simulink model "gm_FP_sub"  (R2023a)
settings: Solver=FixedStepAuto  StartTime=0.0  StopTime=T  RelTol=1e-3  EnableMultiTasking=on
undefined symbols (not defined in the file or in its folder): Ts
libraries: My_FI_Operations x114, simulink x1
(part 1 of 2)
settings Model: Creator=kavru  LastModifiedBy=kolbe
settings OptimizationCC: BlockReduction=off  ConditionallyExecuteInputs=off
settings DebuggingCC: SignalRangeChecking=warning  InheritedTsInSrcMsg=none  SingleTaskRateTransMsg=error  UnconnectedInputMsg=warning  UnconnectedOutputMsg=warning  UnconnectedLineMsg=warning
settings ModelReferenceCC: EnableRefExpFcnMdlSchedulingChecks=on
settings RTWCC: DLArmComputeVersion=19.05

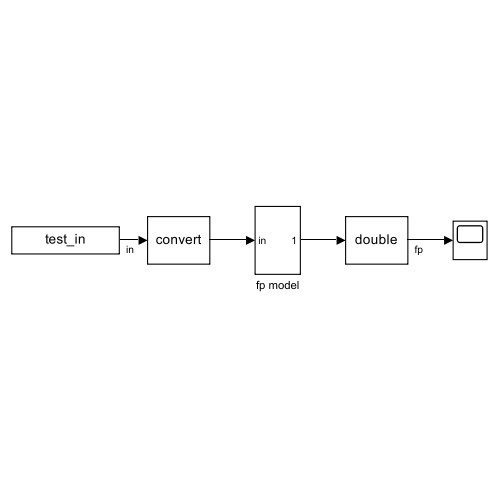
[thumbnail: Simulink's stored preview of the top-level diagram]
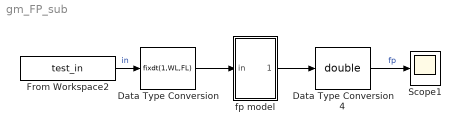
== system gm_FP_sub ==
  Data Type Conversion : DataTypeConversion  OutDataTypeStr=fixdt(1,WL,FL)  RndMeth=Nearest
  Data Type Conversion4 : DataTypeConversion  OutDataTypeStr=double  RndMeth=Nearest  SaturateOnIntegerOverflow=off
  From Workspace2 : FromWorkspace  VariableName=test_in  OutDataTypeStr=double  SampleTime=Ts
  Scope1 : Scope
  fp model : Subsystem
  wires:
  Data Type Conversion4/1 -> Scope1/1  "fp"
  Data Type Conversion/1 -> fp model/1(in)
  fp model/1(Out1) -> Data Type Conversion4/1
  From Workspace2/1 -> Data Type Conversion/1  "in"

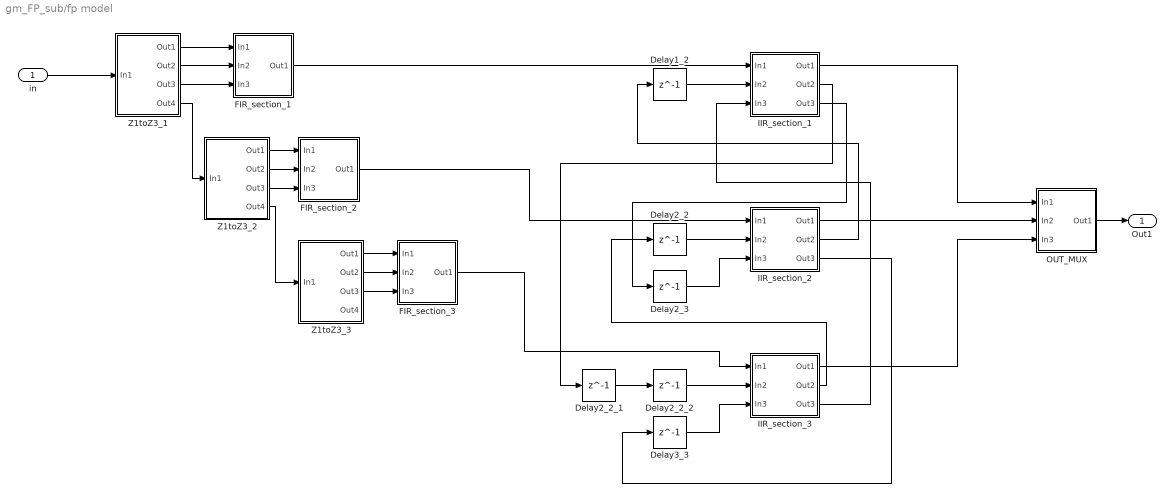
== system gm_FP_sub/fp model ==
  in : Inport
  Delay1_2 : Delay  DelayLength=1  SampleTime=3*Ts
  Delay2_2 : Delay  DelayLength=1  SampleTime=3*Ts
  Delay2_2_1 : Delay  DelayLength=1  SampleTime=3*Ts
  Delay2_2_2 : Delay  DelayLength=1  SampleTime=3*Ts
  Delay2_3 : Delay  DelayLength=1  SampleTime=3*Ts
  Delay3_3 : Delay  DelayLength=1  SampleTime=3*Ts
  FIR_section_1 : Subsystem
  FIR_section_2 : Subsystem
  FIR_section_3 : Subsystem
  IIR_section_1 : Subsystem
  IIR_section_2 : Subsystem
  IIR_section_3 : Subsystem
  OUT_MUX : Subsystem
  Z1toZ3_1 : Subsystem
  Z1toZ3_2 : Subsystem
  Z1toZ3_3 : Subsystem
  Out1 : Outport
  wires:
  IIR_section_1/2(Out2) -> Delay2_2_1/1
  Delay2_2_1/1 -> Delay2_2_2/1
  IIR_section_3/2(Out2) -> Delay2_2/1
  IIR_section_3/1(Out1) -> OUT_MUX/3(In3)
  IIR_section_3/3(Out3) -> IIR_section_1/3(In3)
  FIR_section_3/1(Out1) -> IIR_section_3/1(In1)
  Delay3_3/1 -> IIR_section_3/3(In3)
  Delay2_2_2/1 -> IIR_section_3/2(In2)
  IIR_section_2/3(Out3) -> Delay3_3/1
  IIR_section_2/2(Out2) -> Delay1_2/1
  IIR_section_2/1(Out1) -> OUT_MUX/2(In2)
  Delay2_2/1 -> IIR_section_2/2(In2)
  Delay2_3/1 -> IIR_section_2/3(In3)
  FIR_section_2/1(Out1) -> IIR_section_2/1(In1)
  IIR_section_1/3(Out3) -> Delay2_3/1
  IIR_section_1/1(Out1) -> OUT_MUX/1(In1)
  Delay1_2/1 -> IIR_section_1/2(In2)
  FIR_section_1/1(Out1) -> IIR_section_1/1(In1)
  OUT_MUX/1(Out1) -> Out1/1
  Z1toZ3_3/3(Out3) -> FIR_section_3/3(In3)
  Z1toZ3_3/2(Out2) -> FIR_section_3/2(In2)
  Z1toZ3_3/1(Out1) -> FIR_section_3/1(In1)
  Z1toZ3_2/3(Out3) -> FIR_section_2/3(In3)
  Z1toZ3_2/2(Out2) -> FIR_section_2/2(In2)
  Z1toZ3_2/1(Out1) -> FIR_section_2/1(In1)
  Z1toZ3_1/3(Out3) -> FIR_section_1/3(In3)
  Z1toZ3_1/2(Out2) -> FIR_section_1/2(In2)
  Z1toZ3_1/1(Out1) -> FIR_section_1/1(In1)
  Z1toZ3_2/4(Out4) -> Z1toZ3_3/1(In1)
  Z1toZ3_1/4(Out4) -> Z1toZ3_2/1(In1)
  in/1 -> Z1toZ3_1/1(In1)

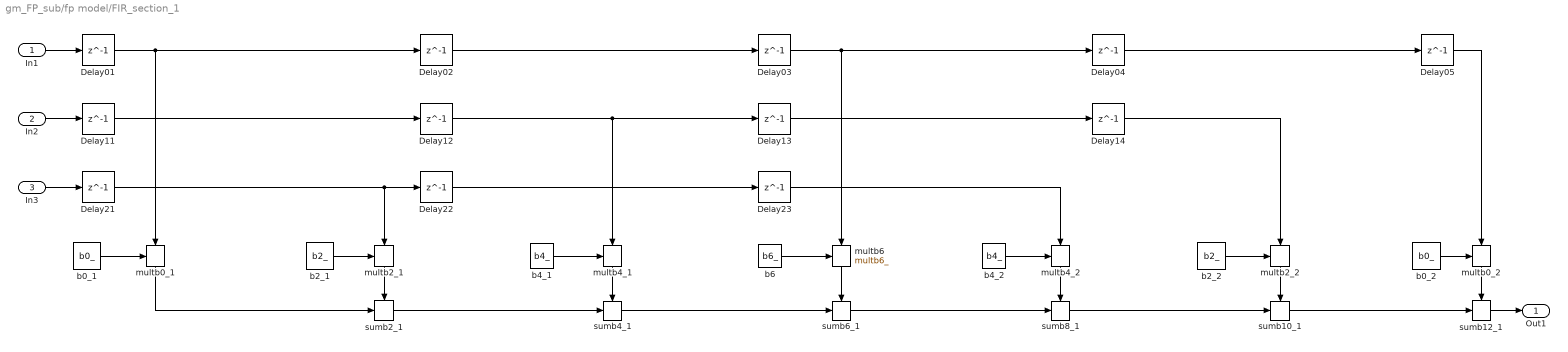
== system gm_FP_sub/fp model/FIR_section_1 ==
  In1 : Inport
  In2 : Inport  Port=2
  In3 : Inport  Port=3
  Delay01 : Delay  DelayLength=1  SampleTime=3*Ts
  Delay02 : Delay  DelayLength=1  SampleTime=3*Ts
  Delay03 : Delay  DelayLength=1  SampleTime=3*Ts
  Delay04 : Delay  DelayLength=1  SampleTime=3*Ts
  Delay05 : Delay  DelayLength=1  SampleTime=3*Ts
  Delay{11..14,21..23} (7 alike) : Delay  DelayLength=1  SampleTime=3*Ts
  b0_1 : My_FI_Operations/b0_  SystemSampleTime=-1  VariantActivationTime=update diagram  Latency=0  AutoFrameSizeCalculation=off
  b0_2 : My_FI_Operations/b0_  SystemSampleTime=-1  VariantActivationTime=update diagram  Latency=0  AutoFrameSizeCalculation=off
  b2_1 : My_FI_Operations/b2_  SystemSampleTime=-1  VariantActivationTime=update diagram  Latency=0  AutoFrameSizeCalculation=off
  b2_2 : My_FI_Operations/b2_  SystemSampleTime=-1  VariantActivationTime=update diagram  Latency=0  AutoFrameSizeCalculation=off
  b4_1 : My_FI_Operations/b4_  SystemSampleTime=-1  VariantActivationTime=update diagram  Latency=0  AutoFrameSizeCalculation=off
  b4_2 : My_FI_Operations/b4_  SystemSampleTime=-1  VariantActivationTime=update diagram  Latency=0  AutoFrameSizeCalculation=off
  b6 : My_FI_Operations/b6_  SystemSampleTime=-1  VariantActivationTime=update diagram  Latency=0  AutoFrameSizeCalculation=off
  multb0_1 : My_FI_Operations/multb0_  SystemSampleTime=-1  VariantActivationTime=update diagram  Latency=0  AutoFrameSizeCalculation=off
      settings: PortSchema="{\"entries\":[{\"content\":{\"sides\":[{\"content\":{\"connectorIds\":[\"In1\"]},\"type\":\"ConnectorPlacement.EquallySpacedRectSide\",\"uuid\":\"20461ecc-945a-453b-bec8-f18bcbd4d7ca\"},{\"content\":{\"connectorIds\":[],\"side\":\"RIGHT\"},\"type\":\"ConnectorPlacement.EquallySpacedRectSide\",\"uuid\":\"a806ae65-26a1-4387-823f-a90265b6c751\"},{\"content\":{\"connectorIds\":[\"In2\"],\"side\":\"TOP\"},\"type\":\"ConnectorPlacement.EquallySpacedRectSide\",\"uuid\":\"faa34e1a-fdc6-4b39-b604-acf00955d353\"},{\"content\":{\"connectorIds\":[\"Out1\"],\"side\":\"BOTTOM\"},\"type\":\"ConnectorPlacement.EquallySpacedRectSide\",\"uuid\":\"6d48c7d1-ec45-4610-bf5d-3af7cf103011\"}]},\"type\":\"ConnectorPlacement.EquallySpacedConnector\",\"uuid\":\"f3c21808-e34e-4785-8275-0070ba5b450f\"}],\"packageUris\":[\"http://schema.mathworks.com/mf0/Connector/R2020b\"],\"version\":\"1.0\"}"
  multb0_2 : My_FI_Operations/multb0_  SystemSampleTime=-1  VariantActivationTime=update diagram  Latency=0  AutoFrameSizeCalculation=off
      settings: PortSchema="{\"entries\":[{\"content\":{\"sides\":[{\"content\":{\"connectorIds\":[\"In1\"]},\"type\":\"ConnectorPlacement.EquallySpacedRectSide\",\"uuid\":\"20461ecc-945a-453b-bec8-f18bcbd4d7ca\"},{\"content\":{\"connectorIds\":[],\"side\":\"RIGHT\"},\"type\":\"ConnectorPlacement.EquallySpacedRectSide\",\"uuid\":\"a806ae65-26a1-4387-823f-a90265b6c751\"},{\"content\":{\"connectorIds\":[\"In2\"],\"side\":\"TOP\"},\"type\":\"ConnectorPlacement.EquallySpacedRectSide\",\"uuid\":\"faa34e1a-fdc6-4b39-b604-acf00955d353\"},{\"content\":{\"connectorIds\":[\"Out1\"],\"side\":\"BOTTOM\"},\"type\":\"ConnectorPlacement.EquallySpacedRectSide\",\"uuid\":\"6d48c7d1-ec45-4610-bf5d-3af7cf103011\"}]},\"type\":\"ConnectorPlacement.EquallySpacedConnector\",\"uuid\":\"f3c21808-e34e-4785-8275-0070ba5b450f\"}],\"packageUris\":[\"http://schema.mathworks.com/mf0/Connector/R2020b\"],\"version\":\"1.0\"}"
  multb2_1 : My_FI_Operations/multb2_  SystemSampleTime=-1  VariantActivationTime=update diagram  Latency=0  AutoFrameSizeCalculation=off
      settings: PortSchema="{\"entries\":[{\"content\":{\"sides\":[{\"content\":{\"connectorIds\":[\"In1\"]},\"type\":\"ConnectorPlacement.EquallySpacedRectSide\",\"uuid\":\"20461ecc-945a-453b-bec8-f18bcbd4d7ca\"},{\"content\":{\"connectorIds\":[],\"side\":\"RIGHT\"},\"type\":\"ConnectorPlacement.EquallySpacedRectSide\",\"uuid\":\"a806ae65-26a1-4387-823f-a90265b6c751\"},{\"content\":{\"connectorIds\":[\"In2\"],\"side\":\"TOP\"},\"type\":\"ConnectorPlacement.EquallySpacedRectSide\",\"uuid\":\"faa34e1a-fdc6-4b39-b604-acf00955d353\"},{\"content\":{\"connectorIds\":[\"Out1\"],\"side\":\"BOTTOM\"},\"type\":\"ConnectorPlacement.EquallySpacedRectSide\",\"uuid\":\"e1b0fef8-c153-494e-8ffe-3515e962a3c5\"}]},\"type\":\"ConnectorPlacement.EquallySpacedConnector\",\"uuid\":\"f3c21808-e34e-4785-8275-0070ba5b450f\"}],\"packageUris\":[\"http://schema.mathworks.com/mf0/Connector/R2020b\"],\"version\":\"1.0\"}"
  multb2_2 : My_FI_Operations/multb2_  SystemSampleTime=-1  VariantActivationTime=update diagram  Latency=0  AutoFrameSizeCalculation=off
      settings: PortSchema="{\"entries\":[{\"content\":{\"sides\":[{\"content\":{\"connectorIds\":[\"In1\"]},\"type\":\"ConnectorPlacement.EquallySpacedRectSide\",\"uuid\":\"20461ecc-945a-453b-bec8-f18bcbd4d7ca\"},{\"content\":{\"connectorIds\":[],\"side\":\"RIGHT\"},\"type\":\"ConnectorPlacement.EquallySpacedRectSide\",\"uuid\":\"a806ae65-26a1-4387-823f-a90265b6c751\"},{\"content\":{\"connectorIds\":[\"In2\"],\"side\":\"TOP\"},\"type\":\"ConnectorPlacement.EquallySpacedRectSide\",\"uuid\":\"faa34e1a-fdc6-4b39-b604-acf00955d353\"},{\"content\":{\"connectorIds\":[\"Out1\"],\"side\":\"BOTTOM\"},\"type\":\"ConnectorPlacement.EquallySpacedRectSide\",\"uuid\":\"e1b0fef8-c153-494e-8ffe-3515e962a3c5\"}]},\"type\":\"ConnectorPlacement.EquallySpacedConnector\",\"uuid\":\"f3c21808-e34e-4785-8275-0070ba5b450f\"}],\"packageUris\":[\"http://schema.mathworks.com/mf0/Connector/R2020b\"],\"version\":\"1.0\"}"
  multb4_1 : My_FI_Operations/multb4_  SystemSampleTime=-1  VariantActivationTime=update diagram  Latency=0  AutoFrameSizeCalculation=off
      settings: PortSchema="{\"entries\":[{\"content\":{\"sides\":[{\"content\":{\"connectorIds\":[\"In1\"]},\"type\":\"ConnectorPlacement.EquallySpacedRectSide\",\"uuid\":\"20461ecc-945a-453b-bec8-f18bcbd4d7ca\"},{\"content\":{\"connectorIds\":[],\"side\":\"RIGHT\"},\"type\":\"ConnectorPlacement.EquallySpacedRectSide\",\"uuid\":\"a806ae65-26a1-4387-823f-a90265b6c751\"},{\"content\":{\"connectorIds\":[\"In2\"],\"side\":\"TOP\"},\"type\":\"ConnectorPlacement.EquallySpacedRectSide\",\"uuid\":\"faa34e1a-fdc6-4b39-b604-acf00955d353\"},{\"content\":{\"connectorIds\":[\"Out1\"],\"side\":\"BOTTOM\"},\"type\":\"ConnectorPlacement.EquallySpacedRectSide\",\"uuid\":\"234e609c-6b95-41af-91dd-8a06091f2e10\"}]},\"type\":\"ConnectorPlacement.EquallySpacedConnector\",\"uuid\":\"f3c21808-e34e-4785-8275-0070ba5b450f\"}],\"packageUris\":[\"http://schema.mathworks.com/mf0/Connector/R2020b\"],\"version\":\"1.0\"}"
  multb4_2 : My_FI_Operations/multb4_  SystemSampleTime=-1  VariantActivationTime=update diagram  Latency=0  AutoFrameSizeCalculation=off
      settings: PortSchema="{\"entries\":[{\"content\":{\"sides\":[{\"content\":{\"connectorIds\":[\"In1\"]},\"type\":\"ConnectorPlacement.EquallySpacedRectSide\",\"uuid\":\"20461ecc-945a-453b-bec8-f18bcbd4d7ca\"},{\"content\":{\"connectorIds\":[],\"side\":\"RIGHT\"},\"type\":\"ConnectorPlacement.EquallySpacedRectSide\",\"uuid\":\"a806ae65-26a1-4387-823f-a90265b6c751\"},{\"content\":{\"connectorIds\":[\"In2\"],\"side\":\"TOP\"},\"type\":\"ConnectorPlacement.EquallySpacedRectSide\",\"uuid\":\"faa34e1a-fdc6-4b39-b604-acf00955d353\"},{\"content\":{\"connectorIds\":[\"Out1\"],\"side\":\"BOTTOM\"},\"type\":\"ConnectorPlacement.EquallySpacedRectSide\",\"uuid\":\"234e609c-6b95-41af-91dd-8a06091f2e10\"}]},\"type\":\"ConnectorPlacement.EquallySpacedConnector\",\"uuid\":\"f3c21808-e34e-4785-8275-0070ba5b450f\"}],\"packageUris\":[\"http://schema.mathworks.com/mf0/Connector/R2020b\"],\"version\":\"1.0\"}"
  multb6 : My_FI_Operations/multb6_  SystemSampleTime=-1  VariantActivationTime=update diagram  Latency=0  AutoFrameSizeCalculation=off
      settings: PortSchema="{\"entries\":[{\"content\":{\"sides\":[{\"content\":{\"connectorIds\":[\"In1\"]},\"type\":\"ConnectorPlacement.EquallySpacedRectSide\",\"uuid\":\"20461ecc-945a-453b-bec8-f18bcbd4d7ca\"},{\"content\":{\"connectorIds\":[],\"side\":\"RIGHT\"},\"type\":\"ConnectorPlacement.EquallySpacedRectSide\",\"uuid\":\"a806ae65-26a1-4387-823f-a90265b6c751\"},{\"content\":{\"connectorIds\":[\"In2\"],\"side\":\"TOP\"},\"type\":\"ConnectorPlacement.EquallySpacedRectSide\",\"uuid\":\"faa34e1a-fdc6-4b39-b604-acf00955d353\"},{\"content\":{\"connectorIds\":[\"Out1\"],\"side\":\"BOTTOM\"},\"type\":\"ConnectorPlacement.EquallySpacedRectSide\",\"uuid\":\"31f2fa17-ae8c-4166-97ac-b63529612348\"}]},\"type\":\"ConnectorPlacement.EquallySpacedConnector\",\"uuid\":\"f3c21808-e34e-4785-8275-0070ba5b450f\"}],\"packageUris\":[\"http://schema.mathworks.com/mf0/Connector/R2020b\"],\"version\":\"1.0\"}"
  sumb10_1 : My_FI_Operations/sumb10_  SystemSampleTime=-1  VariantActivationTime=update diagram  Latency=0  AutoFrameSizeCalculation=off
      settings: PortSchema="{\"entries\":[{\"content\":{\"sides\":[{\"content\":{\"connectorIds\":[\"In1\"]},\"type\":\"ConnectorPlacement.EquallySpacedRectSide\",\"uuid\":\"20461ecc-945a-453b-bec8-f18bcbd4d7ca\"},{\"content\":{\"connectorIds\":[\"Out1\"],\"side\":\"RIGHT\"},\"type\":\"ConnectorPlacement.EquallySpacedRectSide\",\"uuid\":\"a806ae65-26a1-4387-823f-a90265b6c751\"},{\"content\":{\"connectorIds\":[\"In2\"],\"side\":\"TOP\"},\"type\":\"ConnectorPlacement.EquallySpacedRectSide\",\"uuid\":\"faa34e1a-fdc6-4b39-b604-acf00955d353\"}]},\"type\":\"ConnectorPlacement.EquallySpacedConnector\",\"uuid\":\"f3c21808-e34e-4785-8275-0070ba5b450f\"}],\"packageUris\":[\"http://schema.mathworks.com/mf0/Connector/R2020b\"],\"version\":\"1.0\"}"
  sumb12_1 : My_FI_Operations/sumb12_  SystemSampleTime=-1  VariantActivationTime=update diagram  Latency=0  AutoFrameSizeCalculation=off
      settings: PortSchema="{\"entries\":[{\"content\":{\"sides\":[{\"content\":{\"connectorIds\":[\"In1\"]},\"type\":\"ConnectorPlacement.EquallySpacedRectSide\",\"uuid\":\"20461ecc-945a-453b-bec8-f18bcbd4d7ca\"},{\"content\":{\"connectorIds\":[\"Out1\"],\"side\":\"RIGHT\"},\"type\":\"ConnectorPlacement.EquallySpacedRectSide\",\"uuid\":\"a806ae65-26a1-4387-823f-a90265b6c751\"},{\"content\":{\"connectorIds\":[\"In2\"],\"side\":\"TOP\"},\"type\":\"ConnectorPlacement.EquallySpacedRectSide\",\"uuid\":\"faa34e1a-fdc6-4b39-b604-acf00955d353\"}]},\"type\":\"ConnectorPlacement.EquallySpacedConnector\",\"uuid\":\"f3c21808-e34e-4785-8275-0070ba5b450f\"}],\"packageUris\":[\"http://schema.mathworks.com/mf0/Connector/R2020b\"],\"version\":\"1.0\"}"
  sumb2_1 : My_FI_Operations/sumb2_  SystemSampleTime=-1  VariantActivationTime=update diagram  Latency=0  AutoFrameSizeCalculation=off
      settings: PortSchema="{\"entries\":[{\"content\":{\"sides\":[{\"content\":{\"connectorIds\":[\"In1\"]},\"type\":\"ConnectorPlacement.EquallySpacedRectSide\",\"uuid\":\"20461ecc-945a-453b-bec8-f18bcbd4d7ca\"},{\"content\":{\"connectorIds\":[\"Out1\"],\"side\":\"RIGHT\"},\"type\":\"ConnectorPlacement.EquallySpacedRectSide\",\"uuid\":\"a806ae65-26a1-4387-823f-a90265b6c751\"},{\"content\":{\"connectorIds\":[\"In2\"],\"side\":\"TOP\"},\"type\":\"ConnectorPlacement.EquallySpacedRectSide\",\"uuid\":\"faa34e1a-fdc6-4b39-b604-acf00955d353\"}]},\"type\":\"ConnectorPlacement.EquallySpacedConnector\",\"uuid\":\"f3c21808-e34e-4785-8275-0070ba5b450f\"}],\"packageUris\":[\"http://schema.mathworks.com/mf0/Connector/R2020b\"],\"version\":\"1.0\"}"
  sumb4_1 : My_FI_Operations/sumb4_  SystemSampleTime=-1  VariantActivationTime=update diagram  Latency=0  AutoFrameSizeCalculation=off
      settings: PortSchema="{\"entries\":[{\"content\":{\"sides\":[{\"content\":{\"connectorIds\":[\"In1\"]},\"type\":\"ConnectorPlacement.EquallySpacedRectSide\",\"uuid\":\"20461ecc-945a-453b-bec8-f18bcbd4d7ca\"},{\"content\":{\"connectorIds\":[\"Out1\"],\"side\":\"RIGHT\"},\"type\":\"ConnectorPlacement.EquallySpacedRectSide\",\"uuid\":\"a806ae65-26a1-4387-823f-a90265b6c751\"},{\"content\":{\"connectorIds\":[\"In2\"],\"side\":\"TOP\"},\"type\":\"ConnectorPlacement.EquallySpacedRectSide\",\"uuid\":\"faa34e1a-fdc6-4b39-b604-acf00955d353\"}]},\"type\":\"ConnectorPlacement.EquallySpacedConnector\",\"uuid\":\"f3c21808-e34e-4785-8275-0070ba5b450f\"}],\"packageUris\":[\"http://schema.mathworks.com/mf0/Connector/R2020b\"],\"version\":\"1.0\"}"
  sumb6_1 : My_FI_Operations/sumb6_  SystemSampleTime=-1  VariantActivationTime=update diagram  Latency=0  AutoFrameSizeCalculation=off
      settings: PortSchema="{\"entries\":[{\"content\":{\"sides\":[{\"content\":{\"connectorIds\":[\"In1\"]},\"type\":\"ConnectorPlacement.EquallySpacedRectSide\",\"uuid\":\"20461ecc-945a-453b-bec8-f18bcbd4d7ca\"},{\"content\":{\"connectorIds\":[\"Out1\"],\"side\":\"RIGHT\"},\"type\":\"ConnectorPlacement.EquallySpacedRectSide\",\"uuid\":\"a806ae65-26a1-4387-823f-a90265b6c751\"},{\"content\":{\"connectorIds\":[\"In2\"],\"side\":\"TOP\"},\"type\":\"ConnectorPlacement.EquallySpacedRectSide\",\"uuid\":\"faa34e1a-fdc6-4b39-b604-acf00955d353\"}]},\"type\":\"ConnectorPlacement.EquallySpacedConnector\",\"uuid\":\"f3c21808-e34e-4785-8275-0070ba5b450f\"}],\"packageUris\":[\"http://schema.mathworks.com/mf0/Connector/R2020b\"],\"version\":\"1.0\"}"
  sumb8_1 : My_FI_Operations/sumb8_  SystemSampleTime=-1  VariantActivationTime=update diagram  Latency=0  AutoFrameSizeCalculation=off
      settings: PortSchema="{\"entries\":[{\"content\":{\"sides\":[{\"content\":{\"connectorIds\":[\"In1\"]},\"type\":\"ConnectorPlacement.EquallySpacedRectSide\",\"uuid\":\"20461ecc-945a-453b-bec8-f18bcbd4d7ca\"},{\"content\":{\"connectorIds\":[\"Out1\"],\"side\":\"RIGHT\"},\"type\":\"ConnectorPlacement.EquallySpacedRectSide\",\"uuid\":\"a806ae65-26a1-4387-823f-a90265b6c751\"},{\"content\":{\"connectorIds\":[\"In2\"],\"side\":\"TOP\"},\"type\":\"ConnectorPlacement.EquallySpacedRectSide\",\"uuid\":\"faa34e1a-fdc6-4b39-b604-acf00955d353\"}]},\"type\":\"ConnectorPlacement.EquallySpacedConnector\",\"uuid\":\"f3c21808-e34e-4785-8275-0070ba5b450f\"}],\"packageUris\":[\"http://schema.mathworks.com/mf0/Connector/R2020b\"],\"version\":\"1.0\"}"
  Out1 : Outport
  wires:
  In1/1 -> Delay01/1
  sumb10_1/1 -> sumb12_1/1
  Delay04/1 -> Delay05/1
  multb2_2/1 -> sumb10_1/2
  In2/1 -> Delay11/1
  sumb2_1/1 -> sumb4_1/1
  Delay21/1 -> Delay22/1, multb2_1/2
  multb4_2/1 -> sumb8_1/2
  multb0_1/1 -> sumb2_1/1
  multb6/1 -> sumb6_1/2
  sumb12_1/1 -> Out1/1
  b4_1/1 -> multb4_1/1
  b2_1/1 -> multb2_1/1
  Delay05/1 -> multb0_2/2
  b6/1 -> multb6/1
  multb4_1/1 -> sumb4_1/2
  sumb4_1/1 -> sumb6_1/1
  Delay03/1 -> Delay04/1, multb6/2
  Delay02/1 -> Delay03/1
  Delay12/1 -> Delay13/1, multb4_1/2
  multb0_2/1 -> sumb12_1/2
  sumb8_1/1 -> sumb10_1/1
  b4_2/1 -> multb4_2/1
  b0_1/1 -> multb0_1/1
  b0_2/1 -> multb0_2/1
  Delay13/1 -> Delay14/1
  multb2_1/1 -> sumb2_1/2
  sumb6_1/1 -> sumb8_1/1
  Delay23/1 -> multb4_2/2
  b2_2/1 -> multb2_2/1
  Delay22/1 -> Delay23/1
  Delay14/1 -> multb2_2/2
  Delay01/1 -> Delay02/1, multb0_1/2
  Delay11/1 -> Delay12/1
  In3/1 -> Delay21/1

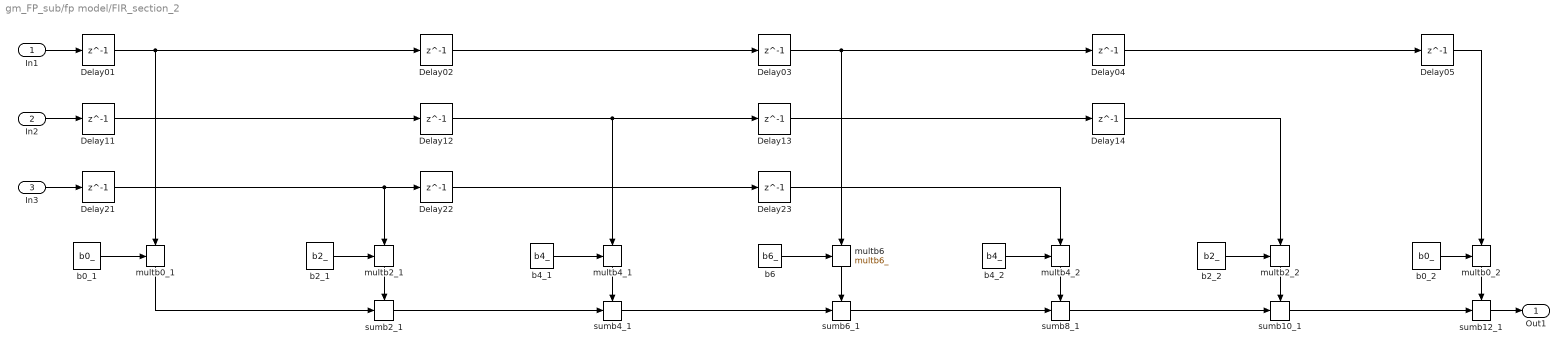
== system gm_FP_sub/fp model/FIR_section_2 ==
  In1 : Inport
  In2 : Inport  Port=2
  In3 : Inport  Port=3
  Delay01 : Delay  DelayLength=1  SampleTime=3*Ts
  Delay02 : Delay  DelayLength=1  SampleTime=3*Ts
  Delay03 : Delay  DelayLength=1  SampleTime=3*Ts
  Delay04 : Delay  DelayLength=1  SampleTime=3*Ts
  Delay05 : Delay  DelayLength=1  SampleTime=3*Ts
  Delay{11..14,21..23} (7 alike) : Delay  DelayLength=1  SampleTime=3*Ts
  b0_1 : My_FI_Operations/b0_  SystemSampleTime=-1  VariantActivationTime=update diagram  Latency=0  AutoFrameSizeCalculation=off
  b0_2 : My_FI_Operations/b0_  SystemSampleTime=-1  VariantActivationTime=update diagram  Latency=0  AutoFrameSizeCalculation=off
  b2_1 : My_FI_Operations/b2_  SystemSampleTime=-1  VariantActivationTime=update diagram  Latency=0  AutoFrameSizeCalculation=off
  b2_2 : My_FI_Operations/b2_  SystemSampleTime=-1  VariantActivationTime=update diagram  Latency=0  AutoFrameSizeCalculation=off
  b4_1 : My_FI_Operations/b4_  SystemSampleTime=-1  VariantActivationTime=update diagram  Latency=0  AutoFrameSizeCalculation=off
  b4_2 : My_FI_Operations/b4_  SystemSampleTime=-1  VariantActivationTime=update diagram  Latency=0  AutoFrameSizeCalculation=off
  b6 : My_FI_Operations/b6_  SystemSampleTime=-1  VariantActivationTime=update diagram  Latency=0  AutoFrameSizeCalculation=off
  multb0_1 : My_FI_Operations/multb0_  SystemSampleTime=-1  VariantActivationTime=update diagram  Latency=0  AutoFrameSizeCalculation=off
      settings: PortSchema="{\"entries\":[{\"content\":{\"sides\":[{\"content\":{\"connectorIds\":[\"In1\"]},\"type\":\"ConnectorPlacement.EquallySpacedRectSide\",\"uuid\":\"20461ecc-945a-453b-bec8-f18bcbd4d7ca\"},{\"content\":{\"connectorIds\":[],\"side\":\"RIGHT\"},\"type\":\"ConnectorPlacement.EquallySpacedRectSide\",\"uuid\":\"a806ae65-26a1-4387-823f-a90265b6c751\"},{\"content\":{\"connectorIds\":[\"In2\"],\"side\":\"TOP\"},\"type\":\"ConnectorPlacement.EquallySpacedRectSide\",\"uuid\":\"faa34e1a-fdc6-4b39-b604-acf00955d353\"},{\"content\":{\"connectorIds\":[\"Out1\"],\"side\":\"BOTTOM\"},\"type\":\"ConnectorPlacement.EquallySpacedRectSide\",\"uuid\":\"6d48c7d1-ec45-4610-bf5d-3af7cf103011\"}]},\"type\":\"ConnectorPlacement.EquallySpacedConnector\",\"uuid\":\"f3c21808-e34e-4785-8275-0070ba5b450f\"}],\"packageUris\":[\"http://schema.mathworks.com/mf0/Connector/R2020b\"],\"version\":\"1.0\"}"
  multb0_2 : My_FI_Operations/multb0_  SystemSampleTime=-1  VariantActivationTime=update diagram  Latency=0  AutoFrameSizeCalculation=off
      settings: PortSchema="{\"entries\":[{\"content\":{\"sides\":[{\"content\":{\"connectorIds\":[\"In1\"]},\"type\":\"ConnectorPlacement.EquallySpacedRectSide\",\"uuid\":\"20461ecc-945a-453b-bec8-f18bcbd4d7ca\"},{\"content\":{\"connectorIds\":[],\"side\":\"RIGHT\"},\"type\":\"ConnectorPlacement.EquallySpacedRectSide\",\"uuid\":\"a806ae65-26a1-4387-823f-a90265b6c751\"},{\"content\":{\"connectorIds\":[\"In2\"],\"side\":\"TOP\"},\"type\":\"ConnectorPlacement.EquallySpacedRectSide\",\"uuid\":\"faa34e1a-fdc6-4b39-b604-acf00955d353\"},{\"content\":{\"connectorIds\":[\"Out1\"],\"side\":\"BOTTOM\"},\"type\":\"ConnectorPlacement.EquallySpacedRectSide\",\"uuid\":\"6d48c7d1-ec45-4610-bf5d-3af7cf103011\"}]},\"type\":\"ConnectorPlacement.EquallySpacedConnector\",\"uuid\":\"f3c21808-e34e-4785-8275-0070ba5b450f\"}],\"packageUris\":[\"http://schema.mathworks.com/mf0/Connector/R2020b\"],\"version\":\"1.0\"}"
  multb2_1 : My_FI_Operations/multb2_  SystemSampleTime=-1  VariantActivationTime=update diagram  Latency=0  AutoFrameSizeCalculation=off
      settings: PortSchema="{\"entries\":[{\"content\":{\"sides\":[{\"content\":{\"connectorIds\":[\"In1\"]},\"type\":\"ConnectorPlacement.EquallySpacedRectSide\",\"uuid\":\"20461ecc-945a-453b-bec8-f18bcbd4d7ca\"},{\"content\":{\"connectorIds\":[],\"side\":\"RIGHT\"},\"type\":\"ConnectorPlacement.EquallySpacedRectSide\",\"uuid\":\"a806ae65-26a1-4387-823f-a90265b6c751\"},{\"content\":{\"connectorIds\":[\"In2\"],\"side\":\"TOP\"},\"type\":\"ConnectorPlacement.EquallySpacedRectSide\",\"uuid\":\"faa34e1a-fdc6-4b39-b604-acf00955d353\"},{\"content\":{\"connectorIds\":[\"Out1\"],\"side\":\"BOTTOM\"},\"type\":\"ConnectorPlacement.EquallySpacedRectSide\",\"uuid\":\"e1b0fef8-c153-494e-8ffe-3515e962a3c5\"}]},\"type\":\"ConnectorPlacement.EquallySpacedConnector\",\"uuid\":\"f3c21808-e34e-4785-8275-0070ba5b450f\"}],\"packageUris\":[\"http://schema.mathworks.com/mf0/Connector/R2020b\"],\"version\":\"1.0\"}"
  multb2_2 : My_FI_Operations/multb2_  SystemSampleTime=-1  VariantActivationTime=update diagram  Latency=0  AutoFrameSizeCalculation=off
      settings: PortSchema="{\"entries\":[{\"content\":{\"sides\":[{\"content\":{\"connectorIds\":[\"In1\"]},\"type\":\"ConnectorPlacement.EquallySpacedRectSide\",\"uuid\":\"20461ecc-945a-453b-bec8-f18bcbd4d7ca\"},{\"content\":{\"connectorIds\":[],\"side\":\"RIGHT\"},\"type\":\"ConnectorPlacement.EquallySpacedRectSide\",\"uuid\":\"a806ae65-26a1-4387-823f-a90265b6c751\"},{\"content\":{\"connectorIds\":[\"In2\"],\"side\":\"TOP\"},\"type\":\"ConnectorPlacement.EquallySpacedRectSide\",\"uuid\":\"faa34e1a-fdc6-4b39-b604-acf00955d353\"},{\"content\":{\"connectorIds\":[\"Out1\"],\"side\":\"BOTTOM\"},\"type\":\"ConnectorPlacement.EquallySpacedRectSide\",\"uuid\":\"e1b0fef8-c153-494e-8ffe-3515e962a3c5\"}]},\"type\":\"ConnectorPlacement.EquallySpacedConnector\",\"uuid\":\"f3c21808-e34e-4785-8275-0070ba5b450f\"}],\"packageUris\":[\"http://schema.mathworks.com/mf0/Connector/R2020b\"],\"version\":\"1.0\"}"
  multb4_1 : My_FI_Operations/multb4_  SystemSampleTime=-1  VariantActivationTime=update diagram  Latency=0  AutoFrameSizeCalculation=off
      settings: PortSchema="{\"entries\":[{\"content\":{\"sides\":[{\"content\":{\"connectorIds\":[\"In1\"]},\"type\":\"ConnectorPlacement.EquallySpacedRectSide\",\"uuid\":\"20461ecc-945a-453b-bec8-f18bcbd4d7ca\"},{\"content\":{\"connectorIds\":[],\"side\":\"RIGHT\"},\"type\":\"ConnectorPlacement.EquallySpacedRectSide\",\"uuid\":\"a806ae65-26a1-4387-823f-a90265b6c751\"},{\"content\":{\"connectorIds\":[\"In2\"],\"side\":\"TOP\"},\"type\":\"ConnectorPlacement.EquallySpacedRectSide\",\"uuid\":\"faa34e1a-fdc6-4b39-b604-acf00955d353\"},{\"content\":{\"connectorIds\":[\"Out1\"],\"side\":\"BOTTOM\"},\"type\":\"ConnectorPlacement.EquallySpacedRectSide\",\"uuid\":\"234e609c-6b95-41af-91dd-8a06091f2e10\"}]},\"type\":\"ConnectorPlacement.EquallySpacedConnector\",\"uuid\":\"f3c21808-e34e-4785-8275-0070ba5b450f\"}],\"packageUris\":[\"http://schema.mathworks.com/mf0/Connector/R2020b\"],\"version\":\"1.0\"}"
  multb4_2 : My_FI_Operations/multb4_  SystemSampleTime=-1  VariantActivationTime=update diagram  Latency=0  AutoFrameSizeCalculation=off
      settings: PortSchema="{\"entries\":[{\"content\":{\"sides\":[{\"content\":{\"connectorIds\":[\"In1\"]},\"type\":\"ConnectorPlacement.EquallySpacedRectSide\",\"uuid\":\"20461ecc-945a-453b-bec8-f18bcbd4d7ca\"},{\"content\":{\"connectorIds\":[],\"side\":\"RIGHT\"},\"type\":\"ConnectorPlacement.EquallySpacedRectSide\",\"uuid\":\"a806ae65-26a1-4387-823f-a90265b6c751\"},{\"content\":{\"connectorIds\":[\"In2\"],\"side\":\"TOP\"},\"type\":\"ConnectorPlacement.EquallySpacedRectSide\",\"uuid\":\"faa34e1a-fdc6-4b39-b604-acf00955d353\"},{\"content\":{\"connectorIds\":[\"Out1\"],\"side\":\"BOTTOM\"},\"type\":\"ConnectorPlacement.EquallySpacedRectSide\",\"uuid\":\"234e609c-6b95-41af-91dd-8a06091f2e10\"}]},\"type\":\"ConnectorPlacement.EquallySpacedConnector\",\"uuid\":\"f3c21808-e34e-4785-8275-0070ba5b450f\"}],\"packageUris\":[\"http://schema.mathworks.com/mf0/Connector/R2020b\"],\"version\":\"1.0\"}"
  multb6 : My_FI_Operations/multb6_  SystemSampleTime=-1  VariantActivationTime=update diagram  Latency=0  AutoFrameSizeCalculation=off
      settings: PortSchema="{\"entries\":[{\"content\":{\"sides\":[{\"content\":{\"connectorIds\":[\"In1\"]},\"type\":\"ConnectorPlacement.EquallySpacedRectSide\",\"uuid\":\"20461ecc-945a-453b-bec8-f18bcbd4d7ca\"},{\"content\":{\"connectorIds\":[],\"side\":\"RIGHT\"},\"type\":\"ConnectorPlacement.EquallySpacedRectSide\",\"uuid\":\"a806ae65-26a1-4387-823f-a90265b6c751\"},{\"content\":{\"connectorIds\":[\"In2\"],\"side\":\"TOP\"},\"type\":\"ConnectorPlacement.EquallySpacedRectSide\",\"uuid\":\"faa34e1a-fdc6-4b39-b604-acf00955d353\"},{\"content\":{\"connectorIds\":[\"Out1\"],\"side\":\"BOTTOM\"},\"type\":\"ConnectorPlacement.EquallySpacedRectSide\",\"uuid\":\"31f2fa17-ae8c-4166-97ac-b63529612348\"}]},\"type\":\"ConnectorPlacement.EquallySpacedConnector\",\"uuid\":\"f3c21808-e34e-4785-8275-0070ba5b450f\"}],\"packageUris\":[\"http://schema.mathworks.com/mf0/Connector/R2020b\"],\"version\":\"1.0\"}"
  sumb10_1 : My_FI_Operations/sumb10_  SystemSampleTime=-1  VariantActivationTime=update diagram  Latency=0  AutoFrameSizeCalculation=off
      settings: PortSchema="{\"entries\":[{\"content\":{\"sides\":[{\"content\":{\"connectorIds\":[\"In1\"]},\"type\":\"ConnectorPlacement.EquallySpacedRectSide\",\"uuid\":\"20461ecc-945a-453b-bec8-f18bcbd4d7ca\"},{\"content\":{\"connectorIds\":[\"Out1\"],\"side\":\"RIGHT\"},\"type\":\"ConnectorPlacement.EquallySpacedRectSide\",\"uuid\":\"a806ae65-26a1-4387-823f-a90265b6c751\"},{\"content\":{\"connectorIds\":[\"In2\"],\"side\":\"TOP\"},\"type\":\"ConnectorPlacement.EquallySpacedRectSide\",\"uuid\":\"faa34e1a-fdc6-4b39-b604-acf00955d353\"}]},\"type\":\"ConnectorPlacement.EquallySpacedConnector\",\"uuid\":\"f3c21808-e34e-4785-8275-0070ba5b450f\"}],\"packageUris\":[\"http://schema.mathworks.com/mf0/Connector/R2020b\"],\"version\":\"1.0\"}"
  sumb12_1 : My_FI_Operations/sumb12_  SystemSampleTime=-1  VariantActivationTime=update diagram  Latency=0  AutoFrameSizeCalculation=off
      settings: PortSchema="{\"entries\":[{\"content\":{\"sides\":[{\"content\":{\"connectorIds\":[\"In1\"]},\"type\":\"ConnectorPlacement.EquallySpacedRectSide\",\"uuid\":\"20461ecc-945a-453b-bec8-f18bcbd4d7ca\"},{\"content\":{\"connectorIds\":[\"Out1\"],\"side\":\"RIGHT\"},\"type\":\"ConnectorPlacement.EquallySpacedRectSide\",\"uuid\":\"a806ae65-26a1-4387-823f-a90265b6c751\"},{\"content\":{\"connectorIds\":[\"In2\"],\"side\":\"TOP\"},\"type\":\"ConnectorPlacement.EquallySpacedRectSide\",\"uuid\":\"faa34e1a-fdc6-4b39-b604-acf00955d353\"}]},\"type\":\"ConnectorPlacement.EquallySpacedConnector\",\"uuid\":\"f3c21808-e34e-4785-8275-0070ba5b450f\"}],\"packageUris\":[\"http://schema.mathworks.com/mf0/Connector/R2020b\"],\"version\":\"1.0\"}"
  sumb2_1 : My_FI_Operations/sumb2_  SystemSampleTime=-1  VariantActivationTime=update diagram  Latency=0  AutoFrameSizeCalculation=off
      settings: PortSchema="{\"entries\":[{\"content\":{\"sides\":[{\"content\":{\"connectorIds\":[\"In1\"]},\"type\":\"ConnectorPlacement.EquallySpacedRectSide\",\"uuid\":\"20461ecc-945a-453b-bec8-f18bcbd4d7ca\"},{\"content\":{\"connectorIds\":[\"Out1\"],\"side\":\"RIGHT\"},\"type\":\"ConnectorPlacement.EquallySpacedRectSide\",\"uuid\":\"a806ae65-26a1-4387-823f-a90265b6c751\"},{\"content\":{\"connectorIds\":[\"In2\"],\"side\":\"TOP\"},\"type\":\"ConnectorPlacement.EquallySpacedRectSide\",\"uuid\":\"faa34e1a-fdc6-4b39-b604-acf00955d353\"}]},\"type\":\"ConnectorPlacement.EquallySpacedConnector\",\"uuid\":\"f3c21808-e34e-4785-8275-0070ba5b450f\"}],\"packageUris\":[\"http://schema.mathworks.com/mf0/Connector/R2020b\"],\"version\":\"1.0\"}"
  sumb4_1 : My_FI_Operations/sumb4_  SystemSampleTime=-1  VariantActivationTime=update diagram  Latency=0  AutoFrameSizeCalculation=off
      settings: PortSchema="{\"entries\":[{\"content\":{\"sides\":[{\"content\":{\"connectorIds\":[\"In1\"]},\"type\":\"ConnectorPlacement.EquallySpacedRectSide\",\"uuid\":\"20461ecc-945a-453b-bec8-f18bcbd4d7ca\"},{\"content\":{\"connectorIds\":[\"Out1\"],\"side\":\"RIGHT\"},\"type\":\"ConnectorPlacement.EquallySpacedRectSide\",\"uuid\":\"a806ae65-26a1-4387-823f-a90265b6c751\"},{\"content\":{\"connectorIds\":[\"In2\"],\"side\":\"TOP\"},\"type\":\"ConnectorPlacement.EquallySpacedRectSide\",\"uuid\":\"faa34e1a-fdc6-4b39-b604-acf00955d353\"}]},\"type\":\"ConnectorPlacement.EquallySpacedConnector\",\"uuid\":\"f3c21808-e34e-4785-8275-0070ba5b450f\"}],\"packageUris\":[\"http://schema.mathworks.com/mf0/Connector/R2020b\"],\"version\":\"1.0\"}"
  sumb6_1 : My_FI_Operations/sumb6_  SystemSampleTime=-1  VariantActivationTime=update diagram  Latency=0  AutoFrameSizeCalculation=off
      settings: PortSchema="{\"entries\":[{\"content\":{\"sides\":[{\"content\":{\"connectorIds\":[\"In1\"]},\"type\":\"ConnectorPlacement.EquallySpacedRectSide\",\"uuid\":\"20461ecc-945a-453b-bec8-f18bcbd4d7ca\"},{\"content\":{\"connectorIds\":[\"Out1\"],\"side\":\"RIGHT\"},\"type\":\"ConnectorPlacement.EquallySpacedRectSide\",\"uuid\":\"a806ae65-26a1-4387-823f-a90265b6c751\"},{\"content\":{\"connectorIds\":[\"In2\"],\"side\":\"TOP\"},\"type\":\"ConnectorPlacement.EquallySpacedRectSide\",\"uuid\":\"faa34e1a-fdc6-4b39-b604-acf00955d353\"}]},\"type\":\"ConnectorPlacement.EquallySpacedConnector\",\"uuid\":\"f3c21808-e34e-4785-8275-0070ba5b450f\"}],\"packageUris\":[\"http://schema.mathworks.com/mf0/Connector/R2020b\"],\"version\":\"1.0\"}"
  sumb8_1 : My_FI_Operations/sumb8_  SystemSampleTime=-1  VariantActivationTime=update diagram  Latency=0  AutoFrameSizeCalculation=off
      settings: PortSchema="{\"entries\":[{\"content\":{\"sides\":[{\"content\":{\"connectorIds\":[\"In1\"]},\"type\":\"ConnectorPlacement.EquallySpacedRectSide\",\"uuid\":\"20461ecc-945a-453b-bec8-f18bcbd4d7ca\"},{\"content\":{\"connectorIds\":[\"Out1\"],\"side\":\"RIGHT\"},\"type\":\"ConnectorPlacement.EquallySpacedRectSide\",\"uuid\":\"a806ae65-26a1-4387-823f-a90265b6c751\"},{\"content\":{\"connectorIds\":[\"In2\"],\"side\":\"TOP\"},\"type\":\"ConnectorPlacement.EquallySpacedRectSide\",\"uuid\":\"faa34e1a-fdc6-4b39-b604-acf00955d353\"}]},\"type\":\"ConnectorPlacement.EquallySpacedConnector\",\"uuid\":\"f3c21808-e34e-4785-8275-0070ba5b450f\"}],\"packageUris\":[\"http://schema.mathworks.com/mf0/Connector/R2020b\"],\"version\":\"1.0\"}"
  Out1 : Outport
  wires:
  In1/1 -> Delay01/1
  sumb10_1/1 -> sumb12_1/1
  Delay04/1 -> Delay05/1
  multb2_2/1 -> sumb10_1/2
  In2/1 -> Delay11/1
  sumb2_1/1 -> sumb4_1/1
  Delay21/1 -> Delay22/1, multb2_1/2
  multb4_2/1 -> sumb8_1/2
  multb0_1/1 -> sumb2_1/1
  multb6/1 -> sumb6_1/2
  sumb12_1/1 -> Out1/1
  b4_1/1 -> multb4_1/1
  b2_1/1 -> multb2_1/1
  Delay05/1 -> multb0_2/2
  b6/1 -> multb6/1
  multb4_1/1 -> sumb4_1/2
  sumb4_1/1 -> sumb6_1/1
  Delay03/1 -> Delay04/1, multb6/2
  Delay02/1 -> Delay03/1
  Delay12/1 -> Delay13/1, multb4_1/2
  multb0_2/1 -> sumb12_1/2
  sumb8_1/1 -> sumb10_1/1
  b4_2/1 -> multb4_2/1
  b0_1/1 -> multb0_1/1
  b0_2/1 -> multb0_2/1
  Delay13/1 -> Delay14/1
  multb2_1/1 -> sumb2_1/2
  sumb6_1/1 -> sumb8_1/1
  Delay23/1 -> multb4_2/2
  b2_2/1 -> multb2_2/1
  Delay22/1 -> Delay23/1
  Delay14/1 -> multb2_2/2
  Delay01/1 -> Delay02/1, multb0_1/2
  Delay11/1 -> Delay12/1
  In3/1 -> Delay21/1

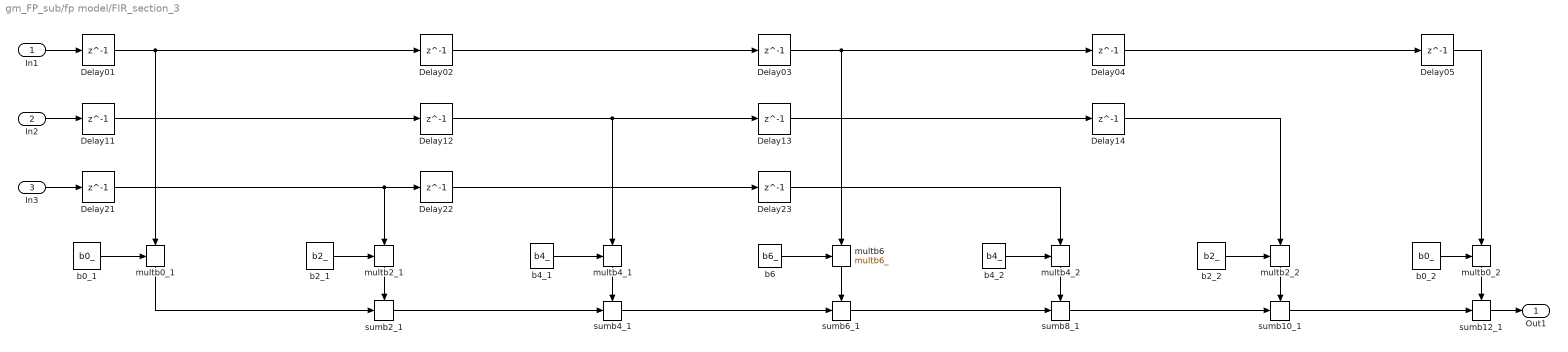
== system gm_FP_sub/fp model/FIR_section_3 ==
  In1 : Inport
  In2 : Inport  Port=2
  In3 : Inport  Port=3
  Delay01 : Delay  DelayLength=1  SampleTime=3*Ts
  Delay02 : Delay  DelayLength=1  SampleTime=3*Ts
  Delay03 : Delay  DelayLength=1  SampleTime=3*Ts
  Delay04 : Delay  DelayLength=1  SampleTime=3*Ts
  Delay05 : Delay  DelayLength=1  SampleTime=3*Ts
  Delay{11..14,21..23} (7 alike) : Delay  DelayLength=1  SampleTime=3*Ts
  b0_1 : My_FI_Operations/b0_  SystemSampleTime=-1  VariantActivationTime=update diagram  Latency=0  AutoFrameSizeCalculation=off
  b0_2 : My_FI_Operations/b0_  SystemSampleTime=-1  VariantActivationTime=update diagram  Latency=0  AutoFrameSizeCalculation=off
  b2_1 : My_FI_Operations/b2_  SystemSampleTime=-1  VariantActivationTime=update diagram  Latency=0  AutoFrameSizeCalculation=off
  b2_2 : My_FI_Operations/b2_  SystemSampleTime=-1  VariantActivationTime=update diagram  Latency=0  AutoFrameSizeCalculation=off
  b4_1 : My_FI_Operations/b4_  SystemSampleTime=-1  VariantActivationTime=update diagram  Latency=0  AutoFrameSizeCalculation=off
  b4_2 : My_FI_Operations/b4_  SystemSampleTime=-1  VariantActivationTime=update diagram  Latency=0  AutoFrameSizeCalculation=off
  b6 : My_FI_Operations/b6_  SystemSampleTime=-1  VariantActivationTime=update diagram  Latency=0  AutoFrameSizeCalculation=off
  multb0_1 : My_FI_Operations/multb0_  SystemSampleTime=-1  VariantActivationTime=update diagram  Latency=0  AutoFrameSizeCalculation=off
      settings: PortSchema="{\"entries\":[{\"content\":{\"sides\":[{\"content\":{\"connectorIds\":[\"In1\"]},\"type\":\"ConnectorPlacement.EquallySpacedRectSide\",\"uuid\":\"20461ecc-945a-453b-bec8-f18bcbd4d7ca\"},{\"content\":{\"connectorIds\":[],\"side\":\"RIGHT\"},\"type\":\"ConnectorPlacement.EquallySpacedRectSide\",\"uuid\":\"a806ae65-26a1-4387-823f-a90265b6c751\"},{\"content\":{\"connectorIds\":[\"In2\"],\"side\":\"TOP\"},\"type\":\"ConnectorPlacement.EquallySpacedRectSide\",\"uuid\":\"faa34e1a-fdc6-4b39-b604-acf00955d353\"},{\"content\":{\"connectorIds\":[\"Out1\"],\"side\":\"BOTTOM\"},\"type\":\"ConnectorPlacement.EquallySpacedRectSide\",\"uuid\":\"6d48c7d1-ec45-4610-bf5d-3af7cf103011\"}]},\"type\":\"ConnectorPlacement.EquallySpacedConnector\",\"uuid\":\"f3c21808-e34e-4785-8275-0070ba5b450f\"}],\"packageUris\":[\"http://schema.mathworks.com/mf0/Connector/R2020b\"],\"version\":\"1.0\"}"
  multb0_2 : My_FI_Operations/multb0_  SystemSampleTime=-1  VariantActivationTime=update diagram  Latency=0  AutoFrameSizeCalculation=off
      settings: PortSchema="{\"entries\":[{\"content\":{\"sides\":[{\"content\":{\"connectorIds\":[\"In1\"]},\"type\":\"ConnectorPlacement.EquallySpacedRectSide\",\"uuid\":\"20461ecc-945a-453b-bec8-f18bcbd4d7ca\"},{\"content\":{\"connectorIds\":[],\"side\":\"RIGHT\"},\"type\":\"ConnectorPlacement.EquallySpacedRectSide\",\"uuid\":\"a806ae65-26a1-4387-823f-a90265b6c751\"},{\"content\":{\"connectorIds\":[\"In2\"],\"side\":\"TOP\"},\"type\":\"ConnectorPlacement.EquallySpacedRectSide\",\"uuid\":\"faa34e1a-fdc6-4b39-b604-acf00955d353\"},{\"content\":{\"connectorIds\":[\"Out1\"],\"side\":\"BOTTOM\"},\"type\":\"ConnectorPlacement.EquallySpacedRectSide\",\"uuid\":\"6d48c7d1-ec45-4610-bf5d-3af7cf103011\"}]},\"type\":\"ConnectorPlacement.EquallySpacedConnector\",\"uuid\":\"f3c21808-e34e-4785-8275-0070ba5b450f\"}],\"packageUris\":[\"http://schema.mathworks.com/mf0/Connector/R2020b\"],\"version\":\"1.0\"}"
  multb2_1 : My_FI_Operations/multb2_  SystemSampleTime=-1  VariantActivationTime=update diagram  Latency=0  AutoFrameSizeCalculation=off
      settings: PortSchema="{\"entries\":[{\"content\":{\"sides\":[{\"content\":{\"connectorIds\":[\"In1\"]},\"type\":\"ConnectorPlacement.EquallySpacedRectSide\",\"uuid\":\"20461ecc-945a-453b-bec8-f18bcbd4d7ca\"},{\"content\":{\"connectorIds\":[],\"side\":\"RIGHT\"},\"type\":\"ConnectorPlacement.EquallySpacedRectSide\",\"uuid\":\"a806ae65-26a1-4387-823f-a90265b6c751\"},{\"content\":{\"connectorIds\":[\"In2\"],\"side\":\"TOP\"},\"type\":\"ConnectorPlacement.EquallySpacedRectSide\",\"uuid\":\"faa34e1a-fdc6-4b39-b604-acf00955d353\"},{\"content\":{\"connectorIds\":[\"Out1\"],\"side\":\"BOTTOM\"},\"type\":\"ConnectorPlacement.EquallySpacedRectSide\",\"uuid\":\"e1b0fef8-c153-494e-8ffe-3515e962a3c5\"}]},\"type\":\"ConnectorPlacement.EquallySpacedConnector\",\"uuid\":\"f3c21808-e34e-4785-8275-0070ba5b450f\"}],\"packageUris\":[\"http://schema.mathworks.com/mf0/Connector/R2020b\"],\"version\":\"1.0\"}"
  multb2_2 : My_FI_Operations/multb2_  SystemSampleTime=-1  VariantActivationTime=update diagram  Latency=0  AutoFrameSizeCalculation=off
      settings: PortSchema="{\"entries\":[{\"content\":{\"sides\":[{\"content\":{\"connectorIds\":[\"In1\"]},\"type\":\"ConnectorPlacement.EquallySpacedRectSide\",\"uuid\":\"20461ecc-945a-453b-bec8-f18bcbd4d7ca\"},{\"content\":{\"connectorIds\":[],\"side\":\"RIGHT\"},\"type\":\"ConnectorPlacement.EquallySpacedRectSide\",\"uuid\":\"a806ae65-26a1-4387-823f-a90265b6c751\"},{\"content\":{\"connectorIds\":[\"In2\"],\"side\":\"TOP\"},\"type\":\"ConnectorPlacement.EquallySpacedRectSide\",\"uuid\":\"faa34e1a-fdc6-4b39-b604-acf00955d353\"},{\"content\":{\"connectorIds\":[\"Out1\"],\"side\":\"BOTTOM\"},\"type\":\"ConnectorPlacement.EquallySpacedRectSide\",\"uuid\":\"e1b0fef8-c153-494e-8ffe-3515e962a3c5\"}]},\"type\":\"ConnectorPlacement.EquallySpacedConnector\",\"uuid\":\"f3c21808-e34e-4785-8275-0070ba5b450f\"}],\"packageUris\":[\"http://schema.mathworks.com/mf0/Connector/R2020b\"],\"version\":\"1.0\"}"
  multb4_1 : My_FI_Operations/multb4_  SystemSampleTime=-1  VariantActivationTime=update diagram  Latency=0  AutoFrameSizeCalculation=off
      settings: PortSchema="{\"entries\":[{\"content\":{\"sides\":[{\"content\":{\"connectorIds\":[\"In1\"]},\"type\":\"ConnectorPlacement.EquallySpacedRectSide\",\"uuid\":\"20461ecc-945a-453b-bec8-f18bcbd4d7ca\"},{\"content\":{\"connectorIds\":[],\"side\":\"RIGHT\"},\"type\":\"ConnectorPlacement.EquallySpacedRectSide\",\"uuid\":\"a806ae65-26a1-4387-823f-a90265b6c751\"},{\"content\":{\"connectorIds\":[\"In2\"],\"side\":\"TOP\"},\"type\":\"ConnectorPlacement.EquallySpacedRectSide\",\"uuid\":\"faa34e1a-fdc6-4b39-b604-acf00955d353\"},{\"content\":{\"connectorIds\":[\"Out1\"],\"side\":\"BOTTOM\"},\"type\":\"ConnectorPlacement.EquallySpacedRectSide\",\"uuid\":\"234e609c-6b95-41af-91dd-8a06091f2e10\"}]},\"type\":\"ConnectorPlacement.EquallySpacedConnector\",\"uuid\":\"f3c21808-e34e-4785-8275-0070ba5b450f\"}],\"packageUris\":[\"http://schema.mathworks.com/mf0/Connector/R2020b\"],\"version\":\"1.0\"}"
  multb4_2 : My_FI_Operations/multb4_  SystemSampleTime=-1  VariantActivationTime=update diagram  Latency=0  AutoFrameSizeCalculation=off
      settings: PortSchema="{\"entries\":[{\"content\":{\"sides\":[{\"content\":{\"connectorIds\":[\"In1\"]},\"type\":\"ConnectorPlacement.EquallySpacedRectSide\",\"uuid\":\"20461ecc-945a-453b-bec8-f18bcbd4d7ca\"},{\"content\":{\"connectorIds\":[],\"side\":\"RIGHT\"},\"type\":\"ConnectorPlacement.EquallySpacedRectSide\",\"uuid\":\"a806ae65-26a1-4387-823f-a90265b6c751\"},{\"content\":{\"connectorIds\":[\"In2\"],\"side\":\"TOP\"},\"type\":\"ConnectorPlacement.EquallySpacedRectSide\",\"uuid\":\"faa34e1a-fdc6-4b39-b604-acf00955d353\"},{\"content\":{\"connectorIds\":[\"Out1\"],\"side\":\"BOTTOM\"},\"type\":\"ConnectorPlacement.EquallySpacedRectSide\",\"uuid\":\"234e609c-6b95-41af-91dd-8a06091f2e10\"}]},\"type\":\"ConnectorPlacement.EquallySpacedConnector\",\"uuid\":\"f3c21808-e34e-4785-8275-0070ba5b450f\"}],\"packageUris\":[\"http://schema.mathworks.com/mf0/Connector/R2020b\"],\"version\":\"1.0\"}"
  multb6 : My_FI_Operations/multb6_  SystemSampleTime=-1  VariantActivationTime=update diagram  Latency=0  AutoFrameSizeCalculation=off
      settings: PortSchema="{\"entries\":[{\"content\":{\"sides\":[{\"content\":{\"connectorIds\":[\"In1\"]},\"type\":\"ConnectorPlacement.EquallySpacedRectSide\",\"uuid\":\"20461ecc-945a-453b-bec8-f18bcbd4d7ca\"},{\"content\":{\"connectorIds\":[],\"side\":\"RIGHT\"},\"type\":\"ConnectorPlacement.EquallySpacedRectSide\",\"uuid\":\"a806ae65-26a1-4387-823f-a90265b6c751\"},{\"content\":{\"connectorIds\":[\"In2\"],\"side\":\"TOP\"},\"type\":\"ConnectorPlacement.EquallySpacedRectSide\",\"uuid\":\"faa34e1a-fdc6-4b39-b604-acf00955d353\"},{\"content\":{\"connectorIds\":[\"Out1\"],\"side\":\"BOTTOM\"},\"type\":\"ConnectorPlacement.EquallySpacedRectSide\",\"uuid\":\"31f2fa17-ae8c-4166-97ac-b63529612348\"}]},\"type\":\"ConnectorPlacement.EquallySpacedConnector\",\"uuid\":\"f3c21808-e34e-4785-8275-0070ba5b450f\"}],\"packageUris\":[\"http://schema.mathworks.com/mf0/Connector/R2020b\"],\"version\":\"1.0\"}"
  sumb10_1 : My_FI_Operations/sumb10_  SystemSampleTime=-1  VariantActivationTime=update diagram  Latency=0  AutoFrameSizeCalculation=off
      settings: PortSchema="{\"entries\":[{\"content\":{\"sides\":[{\"content\":{\"connectorIds\":[\"In1\"]},\"type\":\"ConnectorPlacement.EquallySpacedRectSide\",\"uuid\":\"20461ecc-945a-453b-bec8-f18bcbd4d7ca\"},{\"content\":{\"connectorIds\":[\"Out1\"],\"side\":\"RIGHT\"},\"type\":\"ConnectorPlacement.EquallySpacedRectSide\",\"uuid\":\"a806ae65-26a1-4387-823f-a90265b6c751\"},{\"content\":{\"connectorIds\":[\"In2\"],\"side\":\"TOP\"},\"type\":\"ConnectorPlacement.EquallySpacedRectSide\",\"uuid\":\"faa34e1a-fdc6-4b39-b604-acf00955d353\"}]},\"type\":\"ConnectorPlacement.EquallySpacedConnector\",\"uuid\":\"f3c21808-e34e-4785-8275-0070ba5b450f\"}],\"packageUris\":[\"http://schema.mathworks.com/mf0/Connector/R2020b\"],\"version\":\"1.0\"}"
  sumb12_1 : My_FI_Operations/sumb12_  SystemSampleTime=-1  VariantActivationTime=update diagram  Latency=0  AutoFrameSizeCalculation=off
      settings: PortSchema="{\"entries\":[{\"content\":{\"sides\":[{\"content\":{\"connectorIds\":[\"In1\"]},\"type\":\"ConnectorPlacement.EquallySpacedRectSide\",\"uuid\":\"20461ecc-945a-453b-bec8-f18bcbd4d7ca\"},{\"content\":{\"connectorIds\":[\"Out1\"],\"side\":\"RIGHT\"},\"type\":\"ConnectorPlacement.EquallySpacedRectSide\",\"uuid\":\"a806ae65-26a1-4387-823f-a90265b6c751\"},{\"content\":{\"connectorIds\":[\"In2\"],\"side\":\"TOP\"},\"type\":\"ConnectorPlacement.EquallySpacedRectSide\",\"uuid\":\"faa34e1a-fdc6-4b39-b604-acf00955d353\"}]},\"type\":\"ConnectorPlacement.EquallySpacedConnector\",\"uuid\":\"f3c21808-e34e-4785-8275-0070ba5b450f\"}],\"packageUris\":[\"http://schema.mathworks.com/mf0/Connector/R2020b\"],\"version\":\"1.0\"}"
  sumb2_1 : My_FI_Operations/sumb2_  SystemSampleTime=-1  VariantActivationTime=update diagram  Latency=0  AutoFrameSizeCalculation=off
      settings: PortSchema="{\"entries\":[{\"content\":{\"sides\":[{\"content\":{\"connectorIds\":[\"In1\"]},\"type\":\"ConnectorPlacement.EquallySpacedRectSide\",\"uuid\":\"20461ecc-945a-453b-bec8-f18bcbd4d7ca\"},{\"content\":{\"connectorIds\":[\"Out1\"],\"side\":\"RIGHT\"},\"type\":\"ConnectorPlacement.EquallySpacedRectSide\",\"uuid\":\"a806ae65-26a1-4387-823f-a90265b6c751\"},{\"content\":{\"connectorIds\":[\"In2\"],\"side\":\"TOP\"},\"type\":\"ConnectorPlacement.EquallySpacedRectSide\",\"uuid\":\"faa34e1a-fdc6-4b39-b604-acf00955d353\"}]},\"type\":\"ConnectorPlacement.EquallySpacedConnector\",\"uuid\":\"f3c21808-e34e-4785-8275-0070ba5b450f\"}],\"packageUris\":[\"http://schema.mathworks.com/mf0/Connector/R2020b\"],\"version\":\"1.0\"}"
  sumb4_1 : My_FI_Operations/sumb4_  SystemSampleTime=-1  VariantActivationTime=update diagram  Latency=0  AutoFrameSizeCalculation=off
      settings: PortSchema="{\"entries\":[{\"content\":{\"sides\":[{\"content\":{\"connectorIds\":[\"In1\"]},\"type\":\"ConnectorPlacement.EquallySpacedRectSide\",\"uuid\":\"20461ecc-945a-453b-bec8-f18bcbd4d7ca\"},{\"content\":{\"connectorIds\":[\"Out1\"],\"side\":\"RIGHT\"},\"type\":\"ConnectorPlacement.EquallySpacedRectSide\",\"uuid\":\"a806ae65-26a1-4387-823f-a90265b6c751\"},{\"content\":{\"connectorIds\":[\"In2\"],\"side\":\"TOP\"},\"type\":\"ConnectorPlacement.EquallySpacedRectSide\",\"uuid\":\"faa34e1a-fdc6-4b39-b604-acf00955d353\"}]},\"type\":\"ConnectorPlacement.EquallySpacedConnector\",\"uuid\":\"f3c21808-e34e-4785-8275-0070ba5b450f\"}],\"packageUris\":[\"http://schema.mathworks.com/mf0/Connector/R2020b\"],\"version\":\"1.0\"}"
  sumb6_1 : My_FI_Operations/sumb6_  SystemSampleTime=-1  VariantActivationTime=update diagram  Latency=0  AutoFrameSizeCalculation=off
      settings: PortSchema="{\"entries\":[{\"content\":{\"sides\":[{\"content\":{\"connectorIds\":[\"In1\"]},\"type\":\"ConnectorPlacement.EquallySpacedRectSide\",\"uuid\":\"20461ecc-945a-453b-bec8-f18bcbd4d7ca\"},{\"content\":{\"connectorIds\":[\"Out1\"],\"side\":\"RIGHT\"},\"type\":\"ConnectorPlacement.EquallySpacedRectSide\",\"uuid\":\"a806ae65-26a1-4387-823f-a90265b6c751\"},{\"content\":{\"connectorIds\":[\"In2\"],\"side\":\"TOP\"},\"type\":\"ConnectorPlacement.EquallySpacedRectSide\",\"uuid\":\"faa34e1a-fdc6-4b39-b604-acf00955d353\"}]},\"type\":\"ConnectorPlacement.EquallySpacedConnector\",\"uuid\":\"f3c21808-e34e-4785-8275-0070ba5b450f\"}],\"packageUris\":[\"http://schema.mathworks.com/mf0/Connector/R2020b\"],\"version\":\"1.0\"}"
  sumb8_1 : My_FI_Operations/sumb8_  SystemSampleTime=-1  VariantActivationTime=update diagram  Latency=0  AutoFrameSizeCalculation=off
      settings: PortSchema="{\"entries\":[{\"content\":{\"sides\":[{\"content\":{\"connectorIds\":[\"In1\"]},\"type\":\"ConnectorPlacement.EquallySpacedRectSide\",\"uuid\":\"20461ecc-945a-453b-bec8-f18bcbd4d7ca\"},{\"content\":{\"connectorIds\":[\"Out1\"],\"side\":\"RIGHT\"},\"type\":\"ConnectorPlacement.EquallySpacedRectSide\",\"uuid\":\"a806ae65-26a1-4387-823f-a90265b6c751\"},{\"content\":{\"connectorIds\":[\"In2\"],\"side\":\"TOP\"},\"type\":\"ConnectorPlacement.EquallySpacedRectSide\",\"uuid\":\"faa34e1a-fdc6-4b39-b604-acf00955d353\"}]},\"type\":\"ConnectorPlacement.EquallySpacedConnector\",\"uuid\":\"f3c21808-e34e-4785-8275-0070ba5b450f\"}],\"packageUris\":[\"http://schema.mathworks.com/mf0/Connector/R2020b\"],\"version\":\"1.0\"}"
  Out1 : Outport
  wires:
  In1/1 -> Delay01/1
  sumb10_1/1 -> sumb12_1/1
  Delay04/1 -> Delay05/1
  multb2_2/1 -> sumb10_1/2
  In2/1 -> Delay11/1
  sumb2_1/1 -> sumb4_1/1
  Delay21/1 -> Delay22/1, multb2_1/2
  multb4_2/1 -> sumb8_1/2
  multb0_1/1 -> sumb2_1/1
  multb6/1 -> sumb6_1/2
  sumb12_1/1 -> Out1/1
  b4_1/1 -> multb4_1/1
  b2_1/1 -> multb2_1/1
  Delay05/1 -> multb0_2/2
  b6/1 -> multb6/1
  multb4_1/1 -> sumb4_1/2
  sumb4_1/1 -> sumb6_1/1
  Delay03/1 -> Delay04/1, multb6/2
  Delay02/1 -> Delay03/1
  Delay12/1 -> Delay13/1, multb4_1/2
  multb0_2/1 -> sumb12_1/2
  sumb8_1/1 -> sumb10_1/1
  b4_2/1 -> multb4_2/1
  b0_1/1 -> multb0_1/1
  b0_2/1 -> multb0_2/1
  Delay13/1 -> Delay14/1
  multb2_1/1 -> sumb2_1/2
  sumb6_1/1 -> sumb8_1/1
  Delay23/1 -> multb4_2/2
  b2_2/1 -> multb2_2/1
  Delay22/1 -> Delay23/1
  Delay14/1 -> multb2_2/2
  Delay01/1 -> Delay02/1, multb0_1/2
  Delay11/1 -> Delay12/1
  In3/1 -> Delay21/1
